simulink model "ITMBS_LEGO_XY_Coordinates"  (R2023a)
settings: Solver=VariableStepAuto  StartTime=0.0  StopTime=20  RelTol=1e-3
undefined symbols (not defined in the file): sigbuilder_block, x_final, y_final
libraries: legoev3lib x3
settings Model: Creator=manis  LastModifiedBy=manis

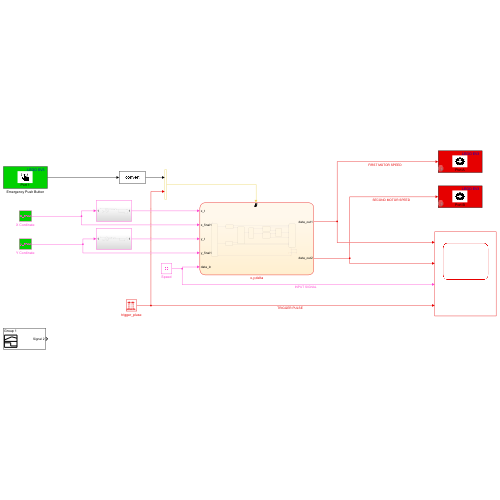
[thumbnail: Simulink's stored preview of the top-level diagram]
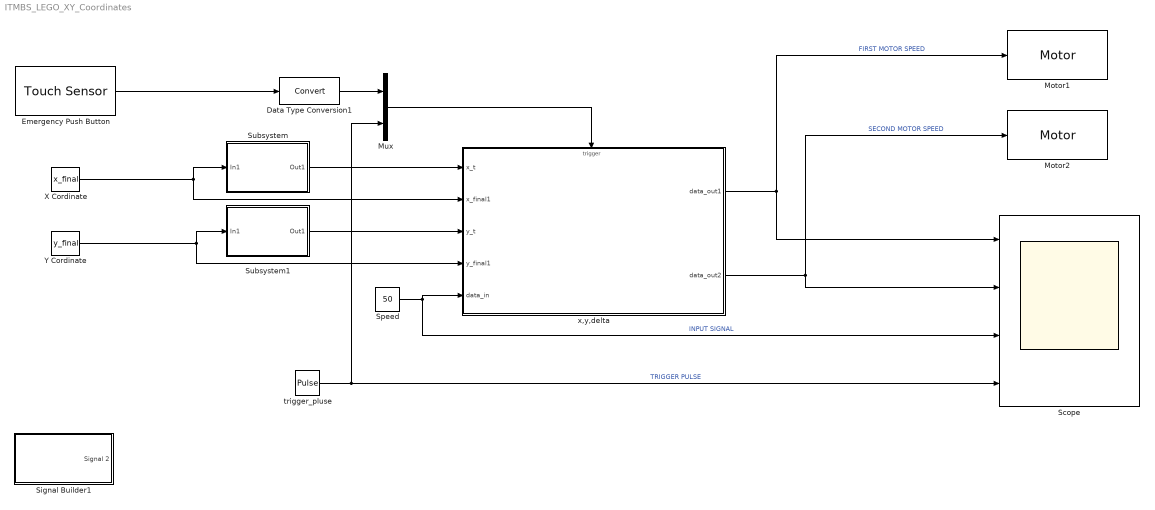
== system ITMBS_LEGO_XY_Coordinates ==
  Data Type Conversion1 : DataTypeConversion  SaturateOnIntegerOverflow=off  RndMeth=Floor
  Emergency Push Button : legoev3lib/Touch Sensor  portNumber=1  sampleTime=0.1
  Motor1 : legoev3lib/Motor  sportNumber=A  sstopAction=Brake
  Motor2 : legoev3lib/Motor  sportNumber=B  sstopAction=Brake
  Mux : Mux  Inputs=2
  Scope : Scope  NumInputPorts=4
  Signal Builder1 : Subsystem  Tag=STV Subsys  LoadFcn=sigbuilder_block('load');  StartFcn=sigbuilder_block('start');  StopFcn=sigbuilder_block('stop');  ClipboardFcn=sigbuilder_block('clipboard');  mask(Sigbuilder block){tuvar=[0:10]}
      mask help: Simulink:masks:SigbuilderBlock_MD
      mask init:
      | if ~strcmp(get_param(bdroot(gcbh),'SimulationStatus'),'stopped') tuvar = sigbuilder_block('maskInit'); end
      settings: CopyFcn=sigbuilder_block('copy');  DeleteFcn=sigbuilder_block('delete');  ModelCloseFcn=sigbuilder_block('modelClose');  PreSaveFcn=sigbuilder_block('preSave');  PauseFcn=sigbuilder_block('pause');  ContinueFcn=sigbuilder_block('continue');  NameChangeFcn=sigbuilder_block('namechange');  OpenFcn=sigbuilder_block('open',[5.4 36 1141.2 516.6 ]);  CloseFcn=sigbuilder_block('close');
      mask Display: plot(0, 0, 100, 100,[2, 2, 32, 32, 2], [68, 8, 8, 68, 68],[32, 2], [38, 38], [32, 19, 2],[53, 60, 44], [32, 17, 17, 2],[16, 16, 31, 31]);txt = getActiveGroup(gcbh);text(2, 100, txt,'verticalAlignment', 'top');
  Speed : Constant  Value=50
  Subsystem : Subsystem
  Subsystem1 : Subsystem
  X Cordinate : Constant  Value=x_final
  Y Cordinate : Constant  Value=y_final
  trigger_pluse : DiscretePulseGenerator  Period=10  PulseWidth=2  SampleTime=0.05
  x,y,delta : Stateflow chart  TreatAsAtomicUnit=on
  wires:
  Mux/1 -> x,y,delta/Trigger
  X Cordinate/1 -> x,y,delta/2(x_final1), Subsystem/1(In1)
  x,y,delta/1(data_out1) -> Motor1/1, Scope/1  "FIRST MOTOR SPEED"
  trigger_pluse/1 -> Mux/2, Scope/4  "TRIGGER PULSE"
  Speed/1 -> Scope/3, x,y,delta/5(data_in)  "INPUT SIGNAL"
  x,y,delta/2(data_out2) -> Scope/2, Motor2/1  "SECOND MOTOR SPEED"
  Y Cordinate/1 -> x,y,delta/4(y_final1), Subsystem1/1(In1)
  Emergency Push Button/1 -> Data Type Conversion1/1
  Subsystem/1(Out1) -> x,y,delta/1(x_t)
  Subsystem1/1(Out1) -> x,y,delta/3(y_t)
  Data Type Conversion1/1 -> Mux/1

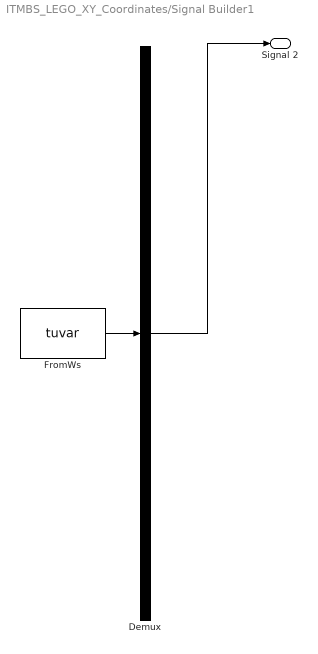
== system ITMBS_LEGO_XY_Coordinates/Signal Builder1 ==
  Demux : Demux  Tag=STV Demux  Outputs=1
      settings: DisplayOption=none
  FromWs : FromWorkspace  Tag=STV FromWs  VariableName=tuvar
      SigBuilderData=|
      | common.afterFinalStr = 'Extrapolate'
      | common.sampleTime = 0
      | dataSet.timeRange = [0 20]
      | dataSet.name = 'Group 1'
      | sbobj.Groups.Name = 'Group 1'
      | sbobj.Groups.Signals.Name = 'Signal 2'
      | sbobj.Groups.Signals.XData = [0 1.18 1.18 1.24 1.24 2.64 2.64 2.7 2.7 2.76 2.76 2.84 2.84 20]
      | sbobj.Groups.Signals.YData = [0 0 4 4 0 0 4 4 0 0 4 4 0 0]
      | sbobj.Groups.TimeRange = [0 20]
  Signal 2 : Outport  Tag=STV Outport
  wires:
  FromWs/1 -> Demux/1
  Demux/1 -> Signal 2/1

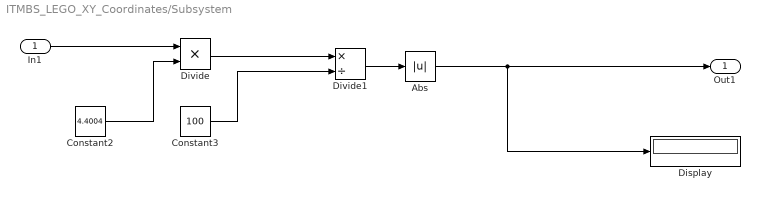
== system ITMBS_LEGO_XY_Coordinates/Subsystem ==
  In1 : Inport
  Abs : Abs  SaturateOnIntegerOverflow=off
  Constant2 : Constant  Value=4.4004
  Constant3 : Constant  Value=100
  Display : Display
  Divide : Product  Inputs=**
  Divide1 : Product  Inputs=*/
  Out1 : Outport
  wires:
  Divide1/1 -> Abs/1
  In1/1 -> Divide/1
  Constant2/1 -> Divide/2
  Divide/1 -> Divide1/1
  Constant3/1 -> Divide1/2
  Abs/1 -> Out1/1, Display/1

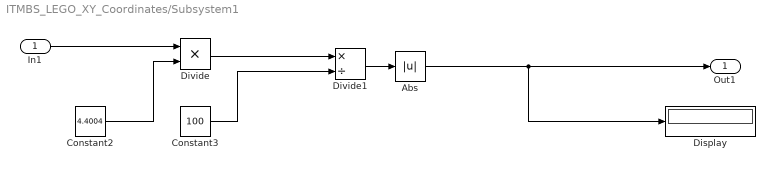
== system ITMBS_LEGO_XY_Coordinates/Subsystem1 ==
  In1 : Inport
  Abs : Abs  SaturateOnIntegerOverflow=off
  Constant2 : Constant  Value=4.4004
  Constant3 : Constant  Value=100
  Display : Display
  Divide : Product  Inputs=**
  Divide1 : Product  Inputs=*/
  Out1 : Outport
  wires:
  Divide1/1 -> Abs/1
  In1/1 -> Divide/1
  Constant2/1 -> Divide/2
  Divide/1 -> Divide1/1
  Constant3/1 -> Divide1/2
  Abs/1 -> Out1/1, Display/1

== stateflow chart ITMBS_LEGO_XY_Coordinates/x,y,delta ==
  state LEGO_Stop1
    data_out1=0;
    data_out2=0;
    entry:
    counter=0;
  state LEGO_90degree_xturn_pos
    data_out1=data_in
    data_out2=0
  state LEGO_break1
    data_out1=0
    data_out2=0
  state LEGO_90degree_yturn_pos
    data_out1=0
    data_out2=data_in
  state LEGO_Run1
    data_out1=data_in
    data_out2=data_in
  state LEGO_break2
    data_out1=0
    data_out2=0
  state LEGO_Run2
    data_out1=data_in
    data_out2=data_in
  state LEGO_90degree_yturn_neg
    data_out1=data_in
    data_out2=0
  state LEGO_Run3
    data_out1=data_in
    data_out2=data_in
  state LEGO_90degree_yturn_pos1
    data_out1=data_in
    data_out2=0
  state LEGO_break3
    data_out1=0
    data_out2=0
  state LEGO_Run4
    data_out1=data_in
    data_out2=data_in
  state LEGO_90degree_yturn_neg1
    data_out1=0
    data_out2=data_in
  state LEGO_90degree_xturn_neg
    data_out1=0
    data_out2=data_in
  (default) -> LEGO_break1
  LEGO_90degree_xturn_pos -> LEGO_Stop1 [order 1] : pb_event
  LEGO_90degree_yturn_pos -> LEGO_Stop1 [order 1] : pb_event
  LEGO_break1 -> LEGO_90degree_xturn_pos [order 1] : [x_final1>0 && after(0.5,sec)]
  LEGO_90degree_xturn_pos -> LEGO_Run1 [order 2] : after(0.75,sec)
  LEGO_break2 -> LEGO_90degree_yturn_pos [order 1] : [y_final1>0 && after(0.5,sec)]
  LEGO_90degree_yturn_pos -> LEGO_Run2 [order 2] : after(0.75,sec)
  LEGO_Run1 -> LEGO_break2 [order 1] : after(x_t,sec)
  LEGO_Run2 -> LEGO_Stop1 : [pb_event || after(y_t,sec)]
  LEGO_break2 -> LEGO_90degree_yturn_neg [order 2] : [y_final1<0 && after(0.5,sec)]
  LEGO_90degree_yturn_neg -> LEGO_Run2 [order 2] : after(0.75,sec)
  LEGO_90degree_yturn_neg -> LEGO_Stop1 [order 1] : pb_event
  LEGO_Run1 -> LEGO_Stop1 [order 2] : pb_event
  LEGO_90degree_yturn_pos1 -> LEGO_Stop1 [order 1] : pb_event
  LEGO_break3 -> LEGO_90degree_yturn_pos1 [order 1] : [y_final1>0 && after(0.5,sec)]
  LEGO_90degree_yturn_pos1 -> LEGO_Run4 [order 2] : after(0.75,sec)
  LEGO_Run4 -> LEGO_Stop1 : pb_event || after(y_t,sec)
  LEGO_Run3 -> LEGO_break3 [order 2] : after(x_t,sec)
  LEGO_break3 -> LEGO_90degree_yturn_neg1 [order 2] : [y_final1<0 && after(0.5,sec)]
  LEGO_90degree_yturn_neg1 -> LEGO_Run4 [order 2] : after(0.75,sec)
  LEGO_90degree_yturn_neg1 -> LEGO_Stop1 [order 1] : pb_event
  LEGO_90degree_xturn_neg -> LEGO_Run3 [order 2] : after(0.75,sec)
  LEGO_Run3 -> LEGO_Stop1 [order 1] : pb_event
  LEGO_break1 -> LEGO_90degree_xturn_neg [order 2] : [x_final1<0 && after(0.5,sec)]
  LEGO_90degree_xturn_neg -> LEGO_Stop1 [order 1] : pb_event
  LEGO_Stop1 -> (junction 227) : %pb_event
  (junction 227) -> (junction 228) [order 1] : [pb_event]
  (junction 227) -> (junction 230) [order 2]
  (junction 228) -> (junction 223) : {counter=counter+1}
  (junction 230) -> (junction 225) [order 2]
  (junction 223) -> (junction 230)
  (junction 230) -> (junction 229) [order 1]
  (junction 229) -> LEGO_break1 : [counter==2]
  data: x_t input; x_final1 input; y_t input; y_final1 input; data_in input; data_out1 output; counter local; data_out2 output; loop local; x_final constant double; y_final constant double
  events: pb_event input RISING_EDGE_EVENT; event input RISING_EDGE_EVENT
